simulink model "faultRecongnize"  (R2016b)
settings: Solver=ode45  StartTime=0  StopTime=0.2  RelTol=1e-3  EnableMultiTasking=on
libraries: powerlib x17
settings Model: Creator=xiang  LastModifiedBy=LiyouWang
settings DataIOCC: LimitDataPoints=on  SaveFormat=Array  SignalLoggingSaveFormat=ModelDataLogs
settings OptimizationCC: ExpressionDepthLimit=2147483647  LifeSpan=inf
settings DebuggingCC: UnderspecifiedInitializationDetection=Classic  MergeDetectMultiDrivingBlocksExec=none  SolverPrmCheckMsg=warning  FcnCallInpInsideContextMsg=warning  StateNameClashWarn=warning  SFUnexpectedBacktrackingDiag=warning  SFNoUnconditionalDefaultTransitionDiag=warning  SFExecutionAtInitializationDiag=none
settings HardwareCC: ProdBitPerPointer=32  ProdBitPerSizeT=32  ProdBitPerPtrDiffT=32  ProdLargestAtomicFloat=None  ProdIntDivRoundTo=Undefined  ProdEndianess=Unspecified  ProdWordSize=32  ProdHWDeviceType=32-bit Generic
settings ModelReferenceCC: PropagateSignalLabelsOutOfModel=off
settings GRTTargetCC: TargetLangStandard=C89/C90 (ANSI)  GeneratePreprocessorConditionals=Disable all
settings ConfigComp: CovMetricSettings=dw  CovHtmlReporting=on  CovSaveCumulativeToWorkspaceVar=on  CovSaveSingleToWorkspaceVar=on  CovExternalEMLEnable=off

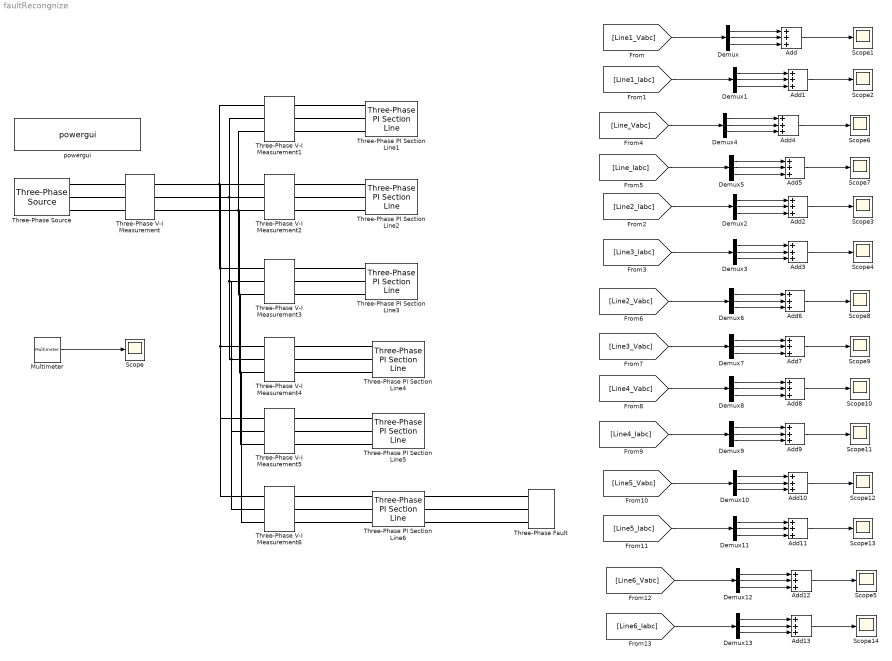
== system faultRecongnize ==
  Add{,1..13} (14 alike) : Sum  Inputs=+++
  Demux{,1..13} (14 alike) : Demux  Outputs=3
  Multimeter : powerlib/Measurements/Multimeter  PhasorSimulation=off  OutputType=Complex  sel=4  L=6  Gain=1  yselected={'Ib: Three-Phase Fault/Fault A'};  PSBOutputType=1  PSBequivalent=0  AxesSetting=[0,0.1,-100,100]  Display=1  SavedBlockNames=-11
  Scope{,1..14} (15 alike) : Scope
  Three-Phase PI Section Line1 : powerlib/Elements/Three-Phase PI Section Line  LConnTagsString=a|b|c  RConnTagsString=A|B|C  Frequency=50  Resistances=[ 0.17 0.23]  Inductances=[1.21e-3 5.48e-3]  Capacitances=[9.7e-9 6e-9]  Length=5
  Three-Phase PI Section Line2 : powerlib/Elements/Three-Phase PI Section Line  LConnTagsString=a|b|c  RConnTagsString=A|B|C  Frequency=50  Resistances=[ 0.17 0.23]  Inductances="[ 1.21e-3  5.48e-3]"  Capacitances=[9.7e-9 6e-9]  Length=10
  Three-Phase PI Section Line3 : powerlib/Elements/Three-Phase PI Section Line  LConnTagsString=a|b|c  RConnTagsString=A|B|C  Frequency=50  Resistances=[ 0.17 0.23]  Inductances="[ 1.21e-3  5.48e-3]"  Capacitances=[9.7e-9 6e-9]  Length=12
  Three-Phase PI Section Line4 : powerlib/Elements/Three-Phase PI Section Line  LConnTagsString=a|b|c  RConnTagsString=A|B|C  Frequency=50  Resistances=[ 0.17 0.23]  Inductances="[ 1.21e-3  5.48e-3]"  Capacitances=[9.7e-9 6e-9]  Length=15
  Three-Phase PI Section Line5 : powerlib/Elements/Three-Phase PI Section Line  LConnTagsString=a|b|c  RConnTagsString=A|B|C  Frequency=50  Resistances=[0.17 0.23]  Inductances="[1.21e-3  5.48e-3]"  Capacitances=[9.7e-9 6e-9]  Length=20
  Three-Phase PI Section Line6 : powerlib/Elements/Three-Phase PI Section Line  LConnTagsString=a|b|c  RConnTagsString=A|B|C  Frequency=50  Resistances=[0.17 0.23]  Inductances="[1.21e-3  5.48e-3]"  Capacitances=[9.7e-9 6e-9]  Length=5
  Three-Phase V-I Measurement : powerlib/Measurements/Three-Phase V-I Measurement  VoltageMeasurement=phase-to-ground  SetLabelV=on  LabelV=Line_Vabc  Vpu=off  VpuLL=off  CurrentMeasurement=yes  SetLabelI=on  LabelI=Line_Iabc  Ipu=off  Pbase=100e6  Vbase=500e3  OutputType=Complex  PhasorSimulation=off  PSBequivalent=0
  Three-Phase V-I Measurement1 : powerlib/Measurements/Three-Phase V-I Measurement  VoltageMeasurement=phase-to-ground  SetLabelV=on  LabelV=Line1_Vabc  Vpu=off  VpuLL=off  CurrentMeasurement=yes  SetLabelI=on  LabelI=Line1_Iabc  Ipu=off  Pbase=100e6  Vbase=500e3  OutputType=Complex  PhasorSimulation=off  PSBequivalent=0
  Three-Phase V-I Measurement2 : powerlib/Measurements/Three-Phase V-I Measurement  VoltageMeasurement=phase-to-ground  SetLabelV=on  LabelV=Line2_Vabc  Vpu=off  VpuLL=off  CurrentMeasurement=yes  SetLabelI=on  LabelI=Line2_Iabc  Ipu=off  Pbase=100e6  Vbase=500e3  OutputType=Complex  PhasorSimulation=off  PSBequivalent=0
  Three-Phase V-I Measurement3 : powerlib/Measurements/Three-Phase V-I Measurement  VoltageMeasurement=phase-to-ground  SetLabelV=on  LabelV=Line3_Vabc  Vpu=off  VpuLL=off  CurrentMeasurement=yes  SetLabelI=on  LabelI=Line3_Iabc  Ipu=off  Pbase=100e6  Vbase=500e3  OutputType=Complex  PhasorSimulation=off  PSBequivalent=0
  Three-Phase V-I Measurement4 : powerlib/Measurements/Three-Phase V-I Measurement  VoltageMeasurement=phase-to-ground  SetLabelV=on  LabelV=Line4_Vabc  Vpu=off  VpuLL=off  CurrentMeasurement=yes  SetLabelI=on  LabelI=Line4_Iabc  Ipu=off  Pbase=100e6  Vbase=500e3  OutputType=Complex  PhasorSimulation=off  PSBequivalent=0
  Three-Phase V-I Measurement5 : powerlib/Measurements/Three-Phase V-I Measurement  VoltageMeasurement=phase-to-ground  SetLabelV=on  LabelV=Line5_Vabc  Vpu=off  VpuLL=off  CurrentMeasurement=yes  SetLabelI=on  LabelI=Line5_Iabc  Ipu=off  Pbase=100e6  Vbase=500e3  OutputType=Complex  PhasorSimulation=off  PSBequivalent=0
  Three-Phase V-I Measurement6 : powerlib/Measurements/Three-Phase V-I Measurement  VoltageMeasurement=phase-to-ground  SetLabelV=on  LabelV=Line6_Vabc  Vpu=off  VpuLL=off  CurrentMeasurement=yes  SetLabelI=on  LabelI=Line6_Iabc  Ipu=off  Pbase=100e6  Vbase=500e3  OutputType=Complex  PhasorSimulation=off  PSBequivalent=0
  Three-Phase Fault : powerlib/Elements/Three-Phase Fault  InitialStates=0  FaultA=on  FaultB=off  FaultC=off  GroundFault=on  SwitchTimes=[0.04 1]  External=off  SwitchStatus=NaN  FaultResistance=0.0001  GroundResistance=0.0001  SnubberResistance=1e6  SnubberCapacitance=inf  Measurements=Fault voltages and currents
  Three-Phase Source : powerlib/Electrical Sources/Three-Phase Source  InternalConnection=Y  VoltagePhases=off  Voltage=10e3  PhaseAngle=0  Voltage_phases=[25e3 25e3 25e3]/sqrt(3)  PhaseAngles_phases=[0 -120 +120]  Frequency=50  NonIdealSource=on  SpecifyImpedance=off  Resistance=0.00529  Inductance=0.000140  ShortCircuitLevel=100e6  BaseVoltage=10e3  XRratio=7  BusType=swing  Pref=0  Qref=0  Prefabc=[10e3, 10e3, 10e3]  Qrefabc=[0, 0, 0]  Qmin=-inf  Qmax=inf
  powergui : powerlib/powergui  Priority=1  SimulationMode=Discrete  SolverType=Tustin  SampleTime=1e-5  frequency=60  SPID=off  DisableSnubberDevices=off  DisableRonSwitches=off  DisableVfSwitches=off  SwTol=0  DisplayEquations=off  Interpol=off  ExternalGateDelay=off  methode=off  Ts=0  FunctionMessages=off  echomessages=off  HookPort=off  EnableUseOfTLC=off  x0status=blocks  frequencyindice=50  Pbase=100e6  ErrMax=1e-4  Iterations=50  UnitsV=V  UnitsW=MW  buscounter=0  RestoreLinks=warning  ResistiveCurrentMeasurement=off  Frange=[0:2:500]  Ylog=off  Xlog=on  ShowGrid=off  save=off  variable=ZData  structure=0  ZoomFFT=off  StartTime=0.0  cycles=1  DisplayStyle=1  fundamental=60  FreqAxis=off  MaxFrequency=1000  frequencyindicesteady=1  RmsSteady=1  display=off
  wires:
  Multimeter/1 -> Scope/1
  [Line1_Vabc] -> Demux/1
  Demux/1 -> Add/1
  Demux/2 -> Add/2
  Demux/3 -> Add/3
  Add/1 -> Scope1/1
  [Line1_Iabc] -> Demux1/1
  Demux1/1 -> Add1/1
  Demux1/2 -> Add1/2
  Demux1/3 -> Add1/3
  Add1/1 -> Scope2/1
  Demux2/3 -> Add2/3
  Demux3/3 -> Add3/3
  [Line2_Iabc] -> Demux2/1
  Demux2/1 -> Add2/1
  Demux2/2 -> Add2/2
  Add2/1 -> Scope3/1
  [Line3_Iabc] -> Demux3/1
  Demux3/1 -> Add3/1
  Demux3/2 -> Add3/2
  Add3/1 -> Scope4/1
  [Line_Vabc] -> Demux4/1
  Demux4/1 -> Add4/1
  Demux4/2 -> Add4/2
  Demux4/3 -> Add4/3
  Add4/1 -> Scope6/1
  [Line_Iabc] -> Demux5/1
  Demux5/1 -> Add5/1
  Demux5/2 -> Add5/2
  Demux5/3 -> Add5/3
  Add5/1 -> Scope7/1
  Demux6/3 -> Add6/3
  Demux7/3 -> Add7/3
  [Line2_Vabc] -> Demux6/1
  Demux6/1 -> Add6/1
  Demux6/2 -> Add6/2
  Add6/1 -> Scope8/1
  [Line3_Vabc] -> Demux7/1
  Demux7/1 -> Add7/1
  Demux7/2 -> Add7/2
  Add7/1 -> Scope9/1
  Demux8/3 -> Add8/3
  Demux9/3 -> Add9/3
  [Line4_Vabc] -> Demux8/1
  Demux8/1 -> Add8/1
  Demux8/2 -> Add8/2
  Add8/1 -> Scope10/1
  [Line4_Iabc] -> Demux9/1
  Demux9/1 -> Add9/1
  Demux9/2 -> Add9/2
  Add9/1 -> Scope11/1
  Demux10/3 -> Add10/3
  Demux11/3 -> Add11/3
  [Line5_Vabc] -> Demux10/1
  Demux10/1 -> Add10/1
  Demux10/2 -> Add10/2
  Add10/1 -> Scope12/1
  [Line5_Iabc] -> Demux11/1
  Demux11/1 -> Add11/1
  Demux11/2 -> Add11/2
  Add11/1 -> Scope13/1
  Demux12/3 -> Add12/3
  Demux13/3 -> Add13/3
  [Line6_Vabc] -> Demux12/1
  Demux12/1 -> Add12/1
  Demux12/2 -> Add12/2
  Add12/1 -> Scope5/1
  [Line6_Iabc] -> Demux13/1
  Demux13/1 -> Add13/1
  Demux13/2 -> Add13/2
  Add13/1 -> Scope14/1
  connections:
  Three-Phase V-I Measurement/RConn1 -- Three-Phase Source/RConn1
  Three-Phase V-I Measurement/RConn2 -- Three-Phase Source/RConn2
  Three-Phase V-I Measurement/RConn3 -- Three-Phase Source/RConn3
  Three-Phase V-I Measurement/LConn1 -- Three-Phase V-I Measurement6/RConn1 -- Three-Phase V-I Measurement5/RConn1 -- Three-Phase V-I Measurement4/RConn1 -- Three-Phase V-I Measurement3/RConn1 -- Three-Phase V-I Measurement1/RConn1 -- Three-Phase V-I Measurement2/RConn1
  Three-Phase V-I Measurement/LConn2 -- Three-Phase V-I Measurement6/RConn2 -- Three-Phase V-I Measurement5/RConn2 -- Three-Phase V-I Measurement4/RConn2 -- Three-Phase V-I Measurement3/RConn2 -- Three-Phase V-I Measurement1/RConn2 -- Three-Phase V-I Measurement2/RConn2
  Three-Phase V-I Measurement/LConn3 -- Three-Phase V-I Measurement6/RConn3 -- Three-Phase V-I Measurement5/RConn3 -- Three-Phase V-I Measurement4/RConn3 -- Three-Phase V-I Measurement3/RConn3 -- Three-Phase V-I Measurement1/RConn3 -- Three-Phase V-I Measurement2/RConn3
  Three-Phase V-I Measurement1/LConn1 -- Three-Phase PI Section Line1/LConn1
  Three-Phase V-I Measurement1/LConn2 -- Three-Phase PI Section Line1/LConn2
  Three-Phase V-I Measurement1/LConn3 -- Three-Phase PI Section Line1/LConn3
  Three-Phase V-I Measurement2/LConn1 -- Three-Phase PI Section Line2/LConn1
  Three-Phase V-I Measurement2/LConn2 -- Three-Phase PI Section Line2/LConn2
  Three-Phase V-I Measurement2/LConn3 -- Three-Phase PI Section Line2/LConn3
  Three-Phase V-I Measurement3/LConn1 -- Three-Phase PI Section Line3/LConn1
  Three-Phase V-I Measurement3/LConn2 -- Three-Phase PI Section Line3/LConn2
  Three-Phase PI Section Line3/LConn3 -- Three-Phase V-I Measurement3/LConn3
  Three-Phase V-I Measurement4/LConn1 -- Three-Phase PI Section Line4/LConn1
  Three-Phase V-I Measurement4/LConn2 -- Three-Phase PI Section Line4/LConn2
  Three-Phase V-I Measurement4/LConn3 -- Three-Phase PI Section Line4/LConn3
  Three-Phase PI Section Line5/LConn1 -- Three-Phase V-I Measurement5/LConn1
  Three-Phase PI Section Line5/LConn2 -- Three-Phase V-I Measurement5/LConn2
  Three-Phase PI Section Line5/LConn3 -- Three-Phase V-I Measurement5/LConn3
  Three-Phase PI Section Line6/LConn1 -- Three-Phase V-I Measurement6/LConn1
  Three-Phase PI Section Line6/LConn2 -- Three-Phase V-I Measurement6/LConn2
  Three-Phase PI Section Line6/LConn3 -- Three-Phase V-I Measurement6/LConn3
  Three-Phase Fault/LConn1 -- Three-Phase PI Section Line6/RConn1
  Three-Phase Fault/LConn2 -- Three-Phase PI Section Line6/RConn2
  Three-Phase Fault/LConn3 -- Three-Phase PI Section Line6/RConn3
